simulink model "ChildSafetyMonitoringApp"  (R2022a)
settings: Solver=VariableStepAuto  StartTime=0.0  StopTime=10.0  RelTol=1e-3
undefined symbols (not defined in the file): a, Acceleration_Global, b, Current_Location, Cycle_Orientation_, Emergency_Message, Enter_Your_Initial_Position, lati_intial, locationMap, longi_initial, Orientation_alert, Send_Emergency_Message, Set_Speed_to_Zero, Speed_Alert, Speed_X, Speed_Y, Speed_Z, Stop_Alert
libraries: androiduilib x15, androidsensorlib x5, androidaudiovideolib x2, mspfiltlib x1
settings Model: Creator=nimitt  LastModifiedBy=nimitt

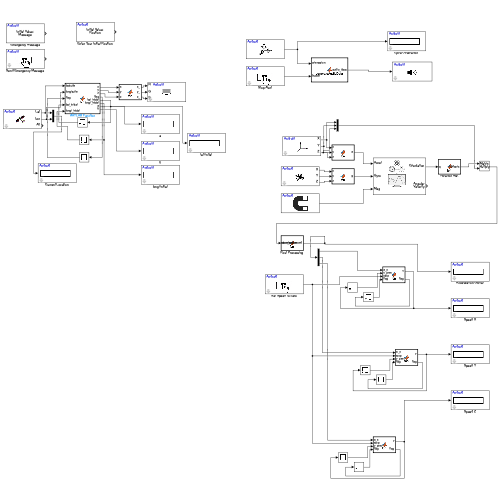
[thumbnail: Simulink's stored preview of the top-level diagram]
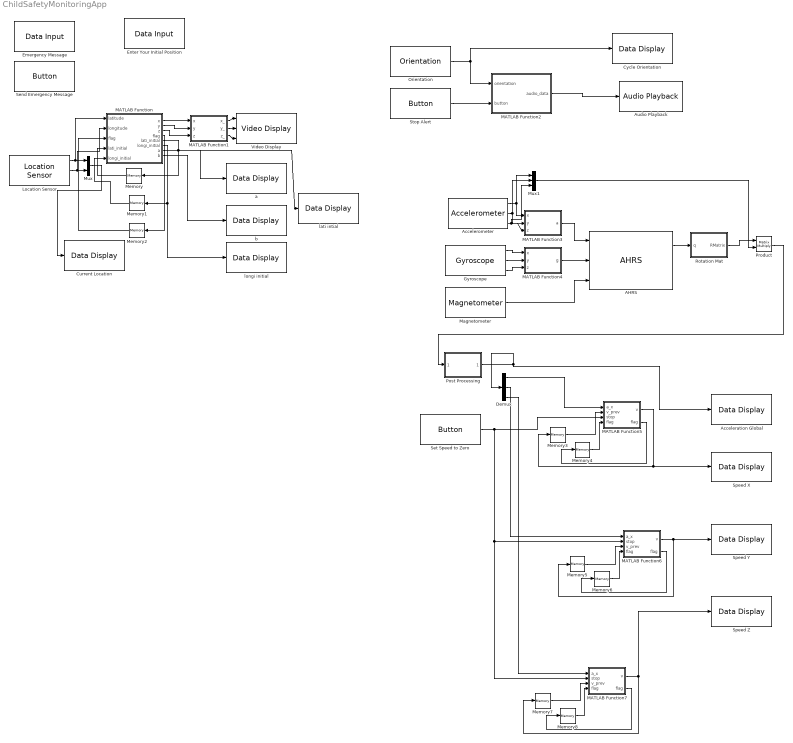
== system ChildSafetyMonitoringApp ==
  AHRS : mspfiltlib/AHRS  DispRefFrame=NED  DecimationFactor=1  InitialProcessNoise=ahrsfilter.defaultProcessNoise  OrientationFormat=quaternion  SimulateUsing=Interpreted execution  AccelerometerNoise=0.0001924722  GyroscopeNoise=9.1385e-5  MagnetometerNoise=0.1  GyroscopeDriftNoise=3.0462e-13  LinearAccelerationNoise=0.0096236100000000012  MagneticDisturbanceNoise=0.5  LinearAccelerationDecayFactor=0.5  MagneticDisturbanceDecayFactor=0.5  ExpectedMagneticFieldStrength=50
      settings: SourceProductBaseCode=NV,TF,NV
  Acceleration Global : androiduilib/Data Display  DataDisplayId=Speed_Alert/Acceleration_Global  Format=Float  Precision=6  SimulateUsing=Code generation  blockPlatform=Android
      settings: SourceProductBaseCode=ANDROID
  Accelerometer : androidsensorlib/Accelerometer  OutputVector=off  SampleTime=0.5  BlockPlatform=Android
      settings: SourceProductBaseCode=ANDROID
  Audio Playback : androidaudiovideolib/Audio Playback  SampleFreq=44100  AudioSamplingFreq=44100  SampleTime=0.1  DeviceStr=0  QueueDuration=0  BlockPlatform=Android
      settings: SourceProductBaseCode=ANDROID
  Current Location : androiduilib/Data Display  DataDisplayId=locationMap/Current_Location  Format=Float  Precision=6  SimulateUsing=Code generation  blockPlatform=Android
      settings: SourceProductBaseCode=ANDROID
  "Cycle Orientation " : androiduilib/Data Display  DataDisplayId=Orientation_alert/Cycle_Orientation_  Format=Float  Precision=6  SimulateUsing=Code generation  blockPlatform=Android
      settings: SourceProductBaseCode=ANDROID
  Demux : Demux  Outputs=3
  Emergency Message : androiduilib/Data Input  isCharVector=on  Value=1.0  CharVector=Message  OutputDataType=double  maxCharVectorSize=255  DataInputId=locationMap/Emergency_Message  SampleTime=0.1
      settings: SourceProductBaseCode=ANDROID
  Enter Your Initial Position : androiduilib/Data Input  isCharVector=on  Value=1.0  CharVector=Position  OutputDataType=double  maxCharVectorSize=255  DataInputId=locationMap/Enter_Your_Initial_Position  SampleTime=0.1
      settings: SourceProductBaseCode=ANDROID
  Gyroscope : androidsensorlib/Gyroscope  OutputVector=off  SampleTime=0.5  BlockPlatform=Android
      settings: SourceProductBaseCode=ANDROID
  Location Sensor : androidsensorlib/Location Sensor  OutputVector=off  SampleTime=0.1  BlockPlatform=Android
      settings: SourceProductBaseCode=ANDROID
  MATLAB Function : MATLAB Function  TreatAsAtomicUnit=on
  MATLAB Function1 : MATLAB Function  TreatAsAtomicUnit=on
  MATLAB Function2 : MATLAB Function  TreatAsAtomicUnit=on
  MATLAB Function3 : MATLAB Function  TreatAsAtomicUnit=on
  MATLAB Function4 : MATLAB Function  TreatAsAtomicUnit=on
  MATLAB Function5 : MATLAB Function  TreatAsAtomicUnit=on
  MATLAB Function6 : MATLAB Function  TreatAsAtomicUnit=on
  MATLAB Function7 : MATLAB Function  TreatAsAtomicUnit=on
  Magnetometer : androidsensorlib/Magnetometer  SampleTime=0.5
      settings: SourceProductBaseCode=ANDROID
  Memory{,1..8} (9 alike) : Memory
  Mux : Mux  Inputs=2
  Mux1 : Mux  Inputs=3
  Orientation : androidsensorlib/Orientation  SampleTime=0.1
      settings: SourceProductBaseCode=ANDROID
  Post Processing : MATLAB Function  TreatAsAtomicUnit=on
  Product : Product  Multiplication=Matrix(*)
  Rotation Mat : MATLAB Function  TreatAsAtomicUnit=on
  Send Emergency Message : androiduilib/Button  ButtonState=Not pressed  ButtonId=locationMap/Send_Emergency_Message  State=off  SampleTime=0.1  BlockPlatform=Android
      settings: SourceProductBaseCode=ANDROID
  Set Speed to Zero : androiduilib/Button  ButtonState=Not pressed  ButtonId=Speed_Alert/Set_Speed_to_Zero  State=off  SampleTime=0.5  BlockPlatform=Android
      settings: SourceProductBaseCode=ANDROID
  Speed X : androiduilib/Data Display  DataDisplayId=Speed_Alert/Speed_X  Format=Float  Precision=6  SimulateUsing=Code generation  blockPlatform=Android
      settings: SourceProductBaseCode=ANDROID
  Speed Y : androiduilib/Data Display  DataDisplayId=Speed_Alert/Speed_Y  Format=Float  Precision=6  SimulateUsing=Code generation  blockPlatform=Android
      settings: SourceProductBaseCode=ANDROID
  Speed Z : androiduilib/Data Display  DataDisplayId=Speed_Alert/Speed_Z  Format=Float  Precision=6  SimulateUsing=Code generation  blockPlatform=Android
      settings: SourceProductBaseCode=ANDROID
  Stop Alert : androiduilib/Button  ButtonState=Not pressed  ButtonId=Orientation_alert/Stop_Alert  State=off  SampleTime=0.1  BlockPlatform=Android
      settings: SourceProductBaseCode=ANDROID
  Video Display : androidaudiovideolib/Video Display  BlockPlatform=Android
      settings: SourceProductBaseCode=ANDROID
  a : androiduilib/Data Display  DataDisplayId=locationMap/a  Format=Float  Precision=6  SimulateUsing=Code generation  blockPlatform=Android
      settings: SourceProductBaseCode=ANDROID
  b : androiduilib/Data Display  DataDisplayId=locationMap/b  Format=Float  Precision=6  SimulateUsing=Code generation  blockPlatform=Android
      settings: SourceProductBaseCode=ANDROID
  lati intial : androiduilib/Data Display  DataDisplayId=locationMap/lati_intial  Format=Float  Precision=6  SimulateUsing=Code generation  blockPlatform=Android
      settings: SourceProductBaseCode=ANDROID
  longi initial : androiduilib/Data Display  DataDisplayId=locationMap/longi_initial  Format=Float  Precision=6  SimulateUsing=Code generation  blockPlatform=Android
      settings: SourceProductBaseCode=ANDROID
  wires:
  Memory1/1 -> MATLAB Function/5("longi_initial ")
  MATLAB Function1/2(y_) -> Video Display/2
  Location Sensor/1 -> MATLAB Function/1(latitude), Mux/1
  Mux/1 -> Current Location/1
  MATLAB Function/4(flag) -> Memory2/1
  MATLAB Function/1(x) -> MATLAB Function1/1(x)
  MATLAB Function/8(b) -> b/1
  MATLAB Function/5(lati_initial) -> lati intial/1, Memory/1
  MATLAB Function/6(longi_initial) -> longi initial/1, Memory1/1
  MATLAB Function1/1(x_) -> Video Display/1
  Location Sensor/2 -> MATLAB Function/2(longitude), Mux/2
  Memory/1 -> MATLAB Function/4("lati_initial ")
  Memory2/1 -> MATLAB Function/3("flag ")
  MATLAB Function1/3(z_) -> Video Display/3
  MATLAB Function/2(y) -> MATLAB Function1/2(y)
  MATLAB Function/3(z) -> MATLAB Function1/3(z)
  MATLAB Function/7(a) -> a/1
  Stop Alert/1 -> MATLAB Function2/2(button)
  Orientation/1 -> "Cycle Orientation "/1, MATLAB Function2/1(orientation)
  MATLAB Function2/1(audio_data) -> Audio Playback/1
  Rotation Mat/1(RMatrix) -> Product/1
  MATLAB Function5/1(v) -> Speed X/1, Memory3/1
  MATLAB Function6/1(v) -> Speed Y/1, Memory5/1
  Set Speed to Zero/1 -> MATLAB Function7/2(stop), MATLAB Function6/2(stop), MATLAB Function5/3(stop)
  Memory3/1 -> MATLAB Function5/2(v_prev)
  Accelerometer/2 -> MATLAB Function3/2(y), Mux1/2
  Demux/3 -> MATLAB Function7/1(a_x)
  MATLAB Function4/1(g) -> AHRS/2
  MATLAB Function5/2(flag) -> Memory4/1
  MATLAB Function7/2(flag) -> Memory8/1
  Accelerometer/3 -> Mux1/3, MATLAB Function3/3(z)
  MATLAB Function6/2(flag) -> Memory6/1
  Demux/2 -> MATLAB Function6/1(a_x)
  Gyroscope/3 -> MATLAB Function4/3(z)
  Memory6/1 -> MATLAB Function6/4("flag ")
  Memory5/1 -> MATLAB Function6/3(v_prev)
  Product/1 -> Post Processing/1(acceleration)
  Memory4/1 -> MATLAB Function5/4("flag ")
  Demux/1 -> MATLAB Function5/1(a_x)
  Mux1/1 -> Product/2
  MATLAB Function3/1(a) -> AHRS/1
  Gyroscope/1 -> MATLAB Function4/1(x)
  Gyroscope/2 -> MATLAB Function4/2(y)
  MATLAB Function7/1(v) -> Speed Z/1, Memory7/1
  Memory7/1 -> MATLAB Function7/3(v_prev)
  Memory8/1 -> MATLAB Function7/4("flag ")
  AHRS/1 -> Rotation Mat/1(q)
  Post Processing/1(acceleration_processed) -> Demux/1, Acceleration Global/1
  Magnetometer/1 -> AHRS/3
  Accelerometer/1 -> Mux1/1, MATLAB Function3/1(x)

== matlab function ChildSafetyMonitoringApp/MATLAB Function7 ==
  data: a_x input; stop input; v output; v_prev input; flag input; flag output
function [v,flag] = fcn(a_x,stop, v_prev,flag)
if (stop)
    flag = 0;
end
if (flag == 0)
v_prev = 0;
flag = 1;
end
dt = 0.5;
v_change = a_x*dt;
v = v_prev + v_change;

== matlab function ChildSafetyMonitoringApp/Post Processing ==
  data: acceleration input; acceleration_processed output
function acceleration_processed = fcn(acceleration)

x = round(acceleration(1));
y = round(acceleration(2));
z = round(acceleration(3))-10;
if abs(x)<2
    x = single(0);
end
if abs(y)<2
    y = single(0);
end
if abs(z)<2
    z = single(0);
end

acceleration_processed = [double(x),double(y),double(z)];

== matlab function ChildSafetyMonitoringApp/Rotation Mat ==
  data: q input; RMatrix output
function RMatrix = fcn(q)
function R = quaternionToRotationMatrix(q)
    q0 = q(1);
    q1 = q(2);
    q2 = q(3);
    q3 = q(4);

    R = [1 - 2*q2^2 - 2*q3^2, 2*q1*q2 - 2*q3*q0, 2*q1*q3 + 2*q2*q0;
         2*q1*q2 + 2*q3*q0, 1 - 2*q1^2 - 2*q3^2, 2*q2*q3 - 2*q1*q0;
         2*q1*q3 - 2*q2*q0, 2*q2*q3 + 2*q1*q0, 1 - 2*q1^2 - 2*q2^2];
end

% Example usage:
% Replace the following line with your quaternion values
RMatrix = quaternionToRotationMatrix(q);
end

== matlab function ChildSafetyMonitoringApp/MATLAB Function1 ==
  data: x input; x_ output; y input; z input; y_ output; z_ output
function [x_,y_,z_] = fcn(x, y, z)
x_ = uint8(x);
y_ = uint8(y);
z_ = uint8(z);

== matlab function ChildSafetyMonitoringApp/MATLAB Function ==
  data: x output; y output; z output; latitude input; longitude input; flag output; flag input; lati_initial input; lati_initial output; longi_initial output; longi_initial input; a output; b output
function [x,y,z,flag,lati_initial,longi_initial,a,b] = fcn(latitude, longitude,flag,lati_initial,longi_initial)

if flag == 0
lati_initial = latitude;
longi_initial = longitude;
flag = 1;
end
% Define image size
imageSize = 1000;

% Create a blank black image
x = (255 * ones(imageSize));
y =(99 * ones(imageSize));
z = (51 * ones(imageSize));

% Define circle parameters
circleCenter = [500, 500];  % Center of the circle (x, y)
circleRadius = 200;         % Radius of the circle

% Create the circle (same code as before)
for i = 1:imageSize
    for j = 1:imageSize
        % Calculate distance from the current pixel to the circle center
        distance = sqrt((i - circleCenter(1))^2 + (j - circleCenter(2))^2);
        
        % Check if the pixel is inside the circle (within the radius)
        if distance <= circleRadius
            % Set pixel values inside the circle to white
            x(i, j) = 208;
            y(i, j) = 255;
            z(i, j) = 51;
        end
    end
end

circleCenter = [500, 500];  % Center of the circle (x, y)
circleRadius = 5;         % Radius of the circle

% Create the circle (same code as before)
for i = 1:imageSize
    for j = 1:imageSize
        % Calculate distance from the current pixel to the circle center
        distance = sqrt((i - circleCenter(1))^2 + (j - circleCenter(2))^2);
        
        % Check if the pixel is inside the circle (within the radius)
        if distance <= circleRadius
            % Set pixel values inside the circle to white
            x(i, j) = 0;
            y(i, j) = 0;
            z(i, j) = 255;
        end
    end
end
% drawing gridlines (same code as before)
for i = 1: 50 : imageSize
for j = 1:imageSize
    x(i, j) = 0;
    y(i, j) = 0;
    z(i, j) = 0;
end
end

for j = 1: 50 : imageSize
for i = 1:imageSize
    x(i, j) = 0;
    y(i, j) = 0;
    z(i, j) = 0;
end
end


a = 500;
b = 500;
a = a + (longitude  - longi_initial)*(20000);
b = b + (latitude - lati_initial)*(20000);

circleCenter = [a, b];  % Center of the circle (x, y)
circleRadius = 5;         % Radius of the circle

% Create the circle (same code as before)
for i = 1:imageSize
    for j = 1:imageSize
        % Calculate distance from the current pixel to the circle center
        distance = sqrt((i - circleCenter(1))^2 + (j - circleCenter(2))^2);
        
        % Check if the pixel is inside the circle (within the radius)
        if distance <= circleRadius
            % Set pixel values inside the circle to white
            x(i, j) = 0;
            y(i, j) = 0;
            z(i, j) = 255;
        end
    end
end

== matlab function ChildSafetyMonitoringApp/MATLAB Function2 ==
  data: audio_data output; orientation input; button input
function audio_data = generateAudioData(orientation, button)
    % Sample audio data generation
    Fs = 4410; % Sampling frequency (Hz)
    t = 0:1/Fs:1-1/Fs; % Time vector (1 second)
    f1 = 440; % Frequency of the left channel (Hz)
    f2 = 880; % Frequency of the right channel (Hz)
    if ((abs(orientation(1)) > 70  || abs(orientation(2)) > 70) && not(button))
        audio_data = [int16(32767*sin(2*pi*f1*t(:))), int16(32767*sin(2*pi*f2*t(:)))];
    else
        audio_data = [int16(0*32767*sin(2*pi*f1*t(:))), int16(0*32767*sin(2*pi*f2*t(:)))];
    end
end

== matlab function ChildSafetyMonitoringApp/MATLAB Function3 ==
  data: x input; a output; y input; z input
function a = fcn(x,y,z)

a = [x,y,z];

== matlab function ChildSafetyMonitoringApp/MATLAB Function4 ==
  data: x input; g output; y input; z input
function g = fcn(x,y,z)

g = [x,y,z];

== matlab function ChildSafetyMonitoringApp/MATLAB Function5 ==
  data: a_x input; v output; v_prev input; stop input; flag input; flag output
function [v,flag] = fcn(a_x,v_prev,stop, flag)
if (stop)
    flag = 0;
end
if (flag == 0)
v_prev = 0;
flag = 1;
end
dt = 0.5;
v_change = a_x*dt;
v = v_prev + v_change;

== matlab function ChildSafetyMonitoringApp/MATLAB Function6 ==
  data: a_x input; stop input; v output; v_prev input; flag input; flag output
function [v,flag] = fcn(a_x,stop, v_prev,flag)
if (stop)
    flag = 0;
end
if (flag == 0)
v_prev = 0;
flag = 1;
end
dt = 0.5;
v_change = a_x*dt;
v = v_prev + v_change;
